simulink model "datascopes"  (R2017a)
settings: Solver=VariableStepAuto  StartTime=0.0  StopTime=250  RelTol=1e-3
settings Model: Creator=user  LastModifiedBy=user

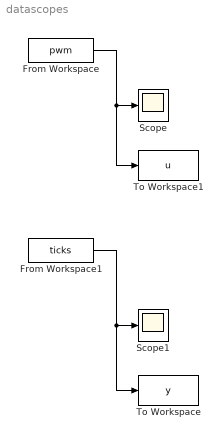
== system datascopes ==
  From Workspace : FromWorkspace  VariableName=pwm  SampleTime=0  Interpolate=off  OutputAfterFinalValue=Holding final value
  From Workspace1 : FromWorkspace  VariableName=ticks  SampleTime=0  Interpolate=off  OutputAfterFinalValue=Holding final value
  Scope : Scope
  Scope1 : Scope
  To Workspace : ToWorkspace  VariableName=y  SaveFormat=Timeseries  SampleTime=-1
  To Workspace1 : ToWorkspace  VariableName=u  SaveFormat=Timeseries  SampleTime=-1
  wires:
  From Workspace/1 -> To Workspace1/1, Scope/1
  From Workspace1/1 -> Scope1/1, To Workspace/1
